simulink model "counter"  (R2018b)
settings: Solver=FixedStepAuto  StartTime=0.0  StopTime=10  RelTol=1e-3
settings Model: Creator=nswat  LastModifiedBy=nswat

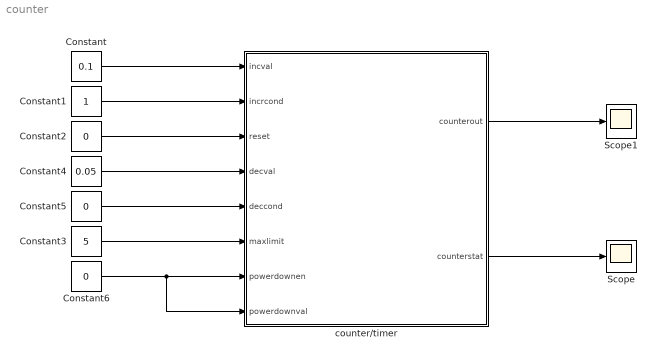
== system counter ==
  Constant : Constant  Value=0.1
  Constant1 : Constant
  Constant2 : Constant  Value=0
  Constant3 : Constant  Value=5
  Constant4 : Constant  Value=0.05
  Constant5 : Constant  Value=0
  Constant6 : Constant  Value=0
  Scope : Scope
  Scope1 : Scope
  counter/timer : Subsystem
  wires:
  Constant/1 -> counter/timer/1(incval)
  Constant1/1 -> counter/timer/2(incrcond)
  Constant2/1 -> counter/timer/3(reset)
  Constant3/1 -> counter/timer/6(maxlimit)
  counter/timer/1(counterout) -> Scope1/1
  counter/timer/2(counterstat) -> Scope/1
  Constant4/1 -> counter/timer/4("decval ")
  Constant5/1 -> counter/timer/5(deccond)
  Constant6/1 -> counter/timer/8(powerdownval), counter/timer/7(powerdownen)

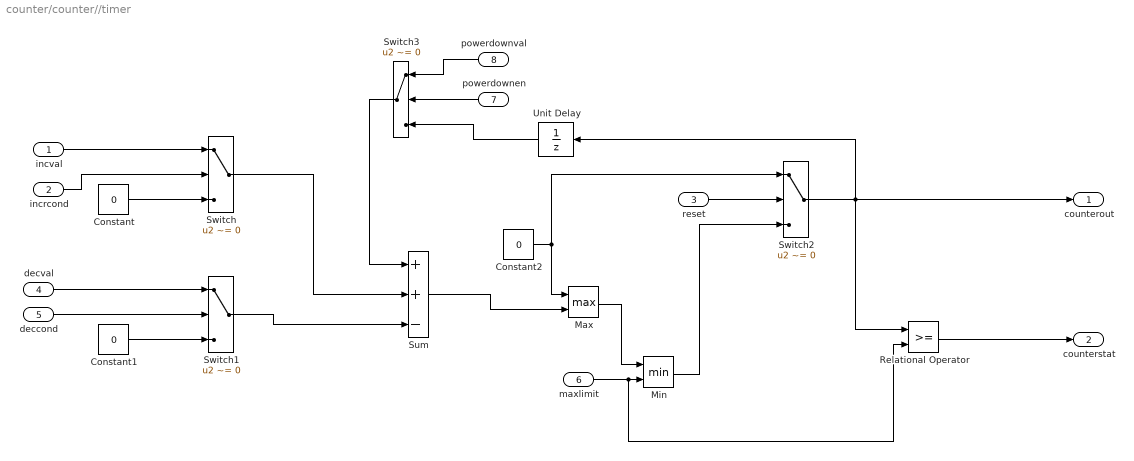
== system counter/counter//timer ==
  incval : Inport
  incrcond : Inport  Port=2
  reset : Inport  Port=3
  "decval " : Inport  Port=4
  deccond : Inport  Port=5
  maxlimit : Inport  Port=6
  powerdownen : Inport  Port=7
  powerdownval : Inport  Port=8
  Constant : Constant  Value=0
  Constant1 : Constant  Value=0
  Constant2 : Constant  Value=0
  Max : MinMax  Function=max  Inputs=2
  Min : MinMax  Inputs=2
  Relational Operator : RelationalOperator  OutDataTypeStr=boolean  RndMeth=Simplest
  Sum : Sum  Inputs=++-
  Switch{,1..3} (4 alike) : Switch  Criteria=u2 ~= 0
  Unit Delay : UnitDelay  SampleTime=-1
  counterout : Outport
  counterstat : Outport  Port=2
  wires:
  Constant1/1 -> Switch1/3
  Switch/1 -> Sum/2
  Switch1/1 -> Sum/3
  reset/1 -> Switch2/2
  Relational Operator/1 -> counterstat/1
  Constant/1 -> Switch/3
  Switch2/1 -> counterout/1, Unit Delay/1, Relational Operator/1
  Sum/1 -> Max/2
  Constant2/1 -> Max/1, Switch2/1
  maxlimit/1 -> Relational Operator/2, Min/2
  incval/1 -> Switch/1
  deccond/1 -> Switch1/2
  "decval "/1 -> Switch1/1
  Max/1 -> Min/1
  incrcond/1 -> Switch/2
  Min/1 -> Switch2/3
  powerdownen/1 -> Switch3/2
  Switch3/1 -> Sum/1
  Unit Delay/1 -> Switch3/3
  powerdownval/1 -> Switch3/1
